simulink model "celsius_TO_fahrenheit"  (R2021a)
settings: Solver=VariableStepAuto  StartTime=0.0  StopTime=10.0  RelTol=1e-3
settings Model: Creator=MAC  LastModifiedBy=MAC

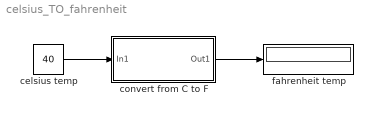
== system celsius_TO_fahrenheit ==
  celsius temp : Constant  Value=40
  convert from C to F : Subsystem
  fahrenheit temp : Display
  wires:
  celsius temp/1 -> convert from C to F/1(In1)
  convert from C to F/1(Out1) -> fahrenheit temp/1

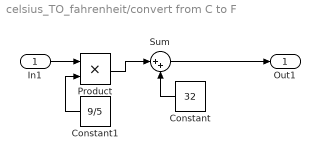
== system celsius_TO_fahrenheit/convert from C to F ==
  In1 : Inport
  Constant : Constant  Value=32
  Constant1 : Constant  Value=9/5
  Product : Product
  Sum : Sum  Inputs=|++
  Out1 : Outport
  wires:
  Sum/1 -> Out1/1
  Constant/1 -> Sum/2
  In1/1 -> Product/1
  Constant1/1 -> Product/2
  Product/1 -> Sum/1
